simulink model "PedalBoardsimulation"  (R2018b)
settings: Solver=FixedStepAuto  StartTime=0.0  StopTime=10.0  RelTol=1e-3
libraries: canoelib x9
settings Model: targetArch=x86  analysisModel=0  XcpMessageLength=-1  hasCAPLCallBlock=0  Creator=jackb  LastModifiedBy=jackb
settings DebuggingCC: LibraryContextMissingDiagnostic=none
settings SFSimCC: SimUseLocalCustomCode=off
settings RTWCC: SystemTargetFile=cn.tlc  TemplateMakefile=cn_msdll.tmf  Description=Vector CANoe Real-Time Target DLL (Visual C/C++ Project Makefile)  RTWUseLocalCustomCode=off
settings STFCustomTargetCC: TargetLangStandard=C99 (ISO)  MatFileLogging=on  GRTInterface=on  SystemTargetFile=cn.tlc
settings GRTTargetCC: ParMdlRefBuildCompliant=off  CompOptLevelCompliant=off  ConcurrentExecutionCompliant=off  CombineOutputUpdateFcns=off  CPPClassGenCompliant=off  GRTInterface=on  UseToolchainInfoCompliant=off
settings ConfigComp: CovEnable=on  RecordCoverage=on  CovModelRefEnable=on

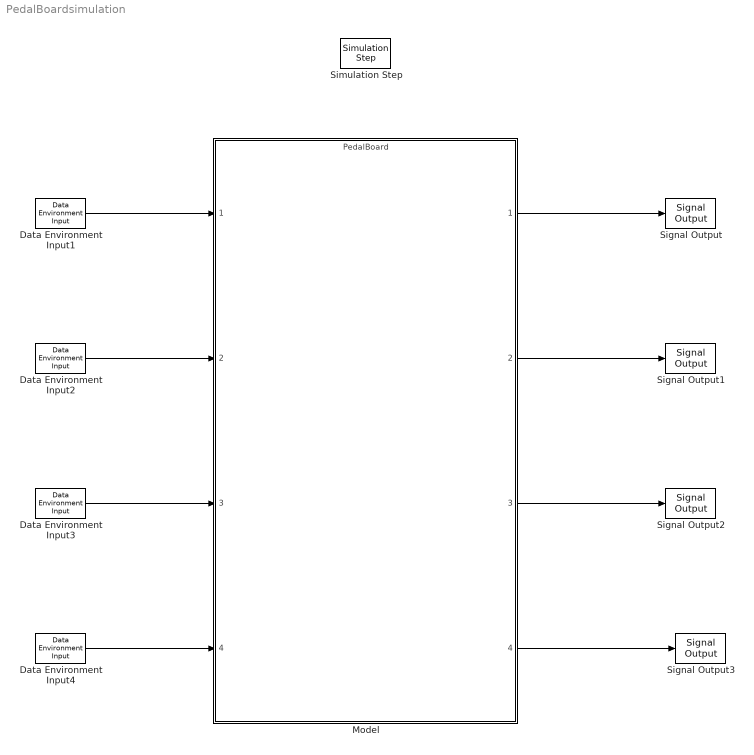
== system PedalBoardsimulation ==
  Data Environment Input1 : canoelib/CANoe I//O/Data Environment Input  envName=Thr_Pos_1  editSampleTime=0  dataType=Default  dataTypeDB=double
      settings: AttributesFormatString=%<envName>  SourceProductName=Vector CANoe
  Data Environment Input2 : canoelib/CANoe I//O/Data Environment Input  envName=Thr_Pos_2  editSampleTime=0  dataType=Default  dataTypeDB=double
      settings: AttributesFormatString=%<envName>  SourceProductName=Vector CANoe
  Data Environment Input3 : canoelib/CANoe I//O/Data Environment Input  envName=Brk_Pos  editSampleTime=0  dataType=Default  dataTypeDB=double
      settings: AttributesFormatString=%<envName>  SourceProductName=Vector CANoe
  Data Environment Input4 : canoelib/CANoe I//O/Data Environment Input  envName=Brk_Ovr_Trv  editSampleTime=0  dataType=Default  dataTypeDB=int32
      settings: AttributesFormatString=%<envName>  SourceProductName=Vector CANoe
  Model : ModelReference  ModelNameDialog=PedalBoard.slx  SimulationMode=Normal  ModelReferenceVersion=1.4
  Signal Output : canoelib/CANoe I//O/Signal Output  dbName=V2CANdb  nodeName=Pedal_Board  msgName=Error_Code  sigName=Error_Code  rawValue=Default  dataType=Default  dataTypeDB=int8  hasEncoding=off
      settings: AttributesFormatString=%<sigName>  SourceProductName=Vector CANoe
  Signal Output1 : canoelib/CANoe I//O/Signal Output  dbName=V2CANdb  nodeName=Pedal_Board  msgName=Pedal_ActualValues  sigName=ped_thr1  rawValue=Default  dataType=Default  dataTypeDB=int8  hasEncoding=off
      settings: AttributesFormatString=%<sigName>  SourceProductName=Vector CANoe
  Signal Output2 : canoelib/CANoe I//O/Signal Output  dbName=V2CANdb  nodeName=Pedal_Board  msgName=Pedal_ActualValues  sigName=ped_brkpos  rawValue=Default  dataType=Default  dataTypeDB=int8  hasEncoding=off
      settings: AttributesFormatString=%<sigName>  SourceProductName=Vector CANoe
  Signal Output3 : canoelib/CANoe I//O/Signal Output  dbName=V2CANdb  nodeName=Pedal_Board  msgName=Pedal_ActualValues  sigName=ped_brkovr  rawValue=Default  dataType=Default  dataTypeDB=int8  hasEncoding=off
      settings: AttributesFormatString=%<sigName>  SourceProductName=Vector CANoe
  Simulation Step : canoelib/CANoe I//O/Simulation Step  mode=Synchronized
      settings: AttributesFormatString=%<mode>  SourceProductName=Vector CANoe
  wires:
  Model/3 -> Signal Output2/1
  Model/4 -> Signal Output3/1
  Model/2 -> Signal Output1/1
  Model/1 -> Signal Output/1
  Data Environment Input4/1 -> Model/4
  Data Environment Input1/1 -> Model/1
  Data Environment Input2/1 -> Model/2
  Data Environment Input3/1 -> Model/3
